simulink model "mconversion15"  (Simulink 8.0)
settings: Solver=FixedStepDiscrete  StartTime=0.0  StopTime=10.0  RelTol=1e-3
settings Model: Creator=awarlock  LastModifiedBy=htu  ExtModeAutoUpdateStatusClock=off
settings DataIOCC: SignalLoggingSaveFormat=ModelDataLogs
settings OptimizationCC: InlineParams=on  InlineInvariantSignals=on  InitFltsAndDblsToZero=on
settings DebuggingCC: SaveWithParameterizedLinksMsg=none  CheckExecutionContextPreStartOutputMsg=on  CheckExecutionContextRuntimeOutputMsg=on  SignalResolutionControl=TryResolveAllWithWarning  MultiTaskDSMMsg=warning  MultiTaskCondExecSysMsg=none
settings RTWCC: IncludeERTFirstTime=on
settings GRTTargetCC: TargetFcnLib=ansi_tfl_tmw.mat  CombineOutputUpdateFcns=off  GRTInterface=on

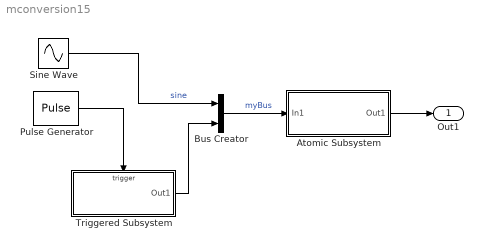
== system mconversion15 ==
  Atomic Subsystem : Subsystem  TreatAsAtomicUnit=on
  Bus Creator : BusCreator  DialogController=Simulink.DDGSource_Bus  Inputs=2
  Pulse Generator : DiscretePulseGenerator  SampleTime=0.1
  Sine Wave : Sin  SampleTime=0.1
  Triggered Subsystem : Subsystem  TreatAsAtomicUnit=on
  Out1 : Outport
  wires:
  Pulse Generator/1 -> Triggered Subsystem/Trigger
  Triggered Subsystem/1(Out1) -> Bus Creator/2
  Bus Creator/1 -> Atomic Subsystem/1(In1)  "myBus"
  Atomic Subsystem/1(Out1) -> Out1/1
  Sine Wave/1 -> Bus Creator/1  "sine"

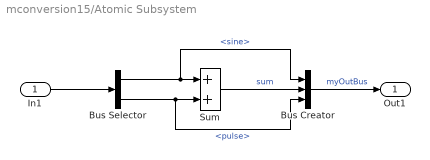
== system mconversion15/Atomic Subsystem ==
  In1 : Inport
  Bus Creator : BusCreator  DialogController=Simulink.DDGSource_Bus  Inputs=3
  Bus Selector : BusSelector  DialogController=Simulink.DDGSource_Bus  OutputSignals=sine,pulse
  Sum : Sum
  Out1 : Outport
  wires:
  In1/1 -> Bus Selector/1
  Bus Selector/1 -> Sum/1, Bus Creator/1  "<sine>"
  Bus Selector/2 -> Sum/2, Bus Creator/3  "<pulse>"
  Sum/1 -> Bus Creator/2  "sum"
  Bus Creator/1 -> Out1/1  "myOutBus"

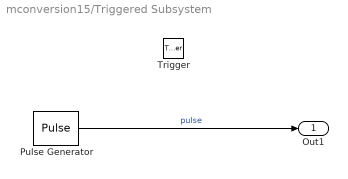
== system mconversion15/Triggered Subsystem ==
  Trigger : TriggerPort
  Pulse Generator : DiscretePulseGenerator  SampleTime=-1
  Out1 : Outport
  wires:
  Pulse Generator/1 -> Out1/1  "pulse"
